simulink model "SolarTrackerVariantSubsystems"  (R2020a)
settings: Solver=FixedStepAuto  StartTime=0.0  StopTime=inf  RelTol=1e-3
model workspace (MAT data in the model file):
  readTSTime = 1
undefined symbols (not defined in the file): Fi, Wi
libraries: sldrtlib x9, arduinowifilib x5, simulink x4, arduinolib x2
settings Model: SILPILModeSetting=veronly  ExtModeTrigDuration=2  Creator=deepakbhatia  LastModifiedBy=cstapels
settings OptimizationCC: EnhancedBackFolding=on  PassReuseOutputArgsAs=Individual arguments  ZeroExternalMemoryAtStartup=off  ZeroInternalMemoryAtStartup=off  MaxStackSize=64  OptimizeBlockOrder=speed  DifferentSizesBufferReuse=on  OptimizationCustomize=off  EfficientTunableParamExpr=on
settings DebuggingCC: ParameterTunabilityLossMsg=error
settings HardwareCC: ProdBitPerPointer=32  ProdBitPerSizeT=32  ProdBitPerPtrDiffT=32  ProdLargestAtomicInteger=Long  ProdLargestAtomicFloat=Double  ProdWordSize=32  ProdHWDeviceType=ARM Compatible->ARM Cortex
settings SFSimCC: MATLABDynamicMemAlloc=off
settings RTWCC: SystemTargetFile=ert.tlc  HardwareBoard=Arduino MKR1000  TLCOptions=-aInlineSetEventsForThisBaseRateFcn=TLC_FALSE -aSuppressMultiTaskScheduler=TLC_FALSE -aRateBasedStepFcn=1  TemplateMakefile=ert_default_tmf  Toolchain=Arduino ARM  BuildConfiguration=Faster Runs
settings CodeAppCC: ForceParamTrailComments=on  IgnoreCustomStorageClasses=off  OperatorAnnotations=on  SimulinkDataObjDesc=on  SFDataObjDesc=on  InsertBlockDesc=on
settings ERTTargetCC: SupportContinuousTime=on  SupportVariableSizeSignals=on  ExtModeStaticAllocSize=8192

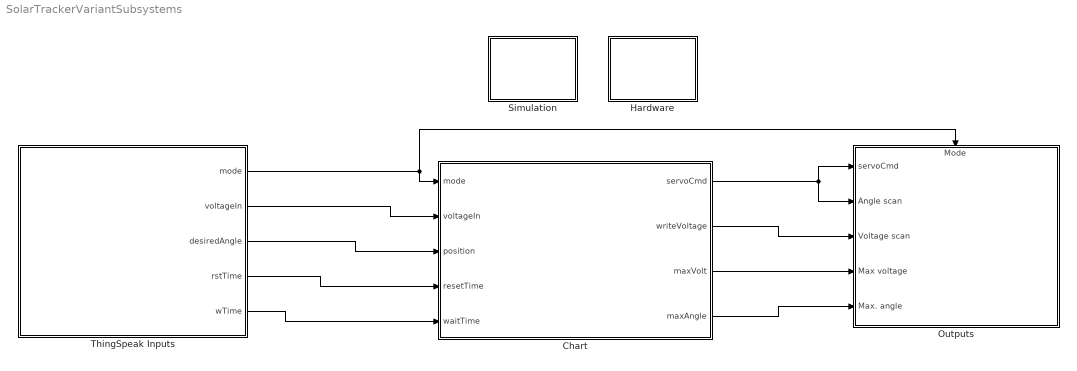
== system SolarTrackerVariantSubsystems ==
  Chart : Stateflow chart  TreatAsAtomicUnit=on
      settings: PortSchema="{\"entries\":[{\"content\":{\"sides\":[{\"content\":{\"connectorIds\":[\"In5\",\"In1\",\"In2\",\"In3\",\"In4\"]},\"type\":\"ConnectorPlacement.EquallySpacedRectSide\",\"uuid\":\"7460febf-f6e8-4dab-9ef6-8acf957c7b17\"},{\"content\":{\"connectorIds\":[\"Out1\",\"Out2\",\"Out3\",\"Out4\"],\"side\":\"RIGHT\"},\"type\":\"ConnectorPlacement.EquallySpacedRectSide\",\"uuid\":\"34f4fde0-3abd-4f83-b5ac-d115b7860e10\"},{\"content\":{\"connectorIds\":[],\"side\":\"TOP\"},\"type\":\"ConnectorPlacement.EquallySpacedRectSide\",\"uuid\":\"03c52414-b361-422d-a974-9760757eaedc\"}]},\"type\":\"ConnectorPlacement.EquallySpacedConnector\",\"uuid\":\"cf5b2fd0-3883-4494-a5b1-8c312db57bd7\"}],\"packageUris\":[\"http://schema.mathworks.com/mf0/Connector/19700101\"],\"version\":\"1.0\"}"
  Hardware : Subsystem
      settings: OpenFcn=|
      | simulationMode = 0
      | model = bdroot;
      | rtwbuild(model)
  Outputs : Subsystem  Variant=on
      settings: PortSchema="{\"entries\":[{\"content\":{\"sides\":[{\"content\":{\"connectorIds\":[\"In1\",\"In2\",\"In3\",\"In4\",\"In5\"]},\"type\":\"ConnectorPlacement.EquallySpacedRectSide\",\"uuid\":\"3daa0852-d339-48d5-aa09-9a267aadeaaa\"},{\"content\":{\"connectorIds\":[],\"side\":\"RIGHT\"},\"type\":\"ConnectorPlacement.EquallySpacedRectSide\",\"uuid\":\"98b05520-bee3-494f-8c4e-0b1eb9c00b10\"},{\"content\":{\"connectorIds\":[\"In6\"],\"side\":\"TOP\"},\"type\":\"ConnectorPlacement.EquallySpacedRectSide\",\"uuid\":\"246e7149-3295-4237-886d-aac11bde170e\"}]},\"type\":\"ConnectorPlacement.EquallySpacedConnector\",\"uuid\":\"0b2c3d1c-3ae1-45ce-8e4d-12c825df3e24\"}],\"packageUris\":[\"http://schema.mathworks.com/mf0/Connector/19700101\"],\"version\":\"1.0\"}"
  Simulation : Subsystem
      settings: OpenFcn=|
      | simulationMode = 1;
      | model=bdroot;
      | set_param(model,'SimulationCommand','start');
  ThingSpeak Inputs : Subsystem  Variant=on
  wires:
  ThingSpeak Inputs/2(voltageIn) -> Chart/1(voltageIn)
  ThingSpeak Inputs/4(rstTime) -> Chart/3(resetTime)
  ThingSpeak Inputs/5(wTime) -> Chart/4(waitTime)
  Chart/4(maxAngle) -> Outputs/5(Max. angle)
  ThingSpeak Inputs/1(mode) -> Chart/5(mode), Outputs/6(Mode)
  Chart/2(writeVoltage) -> Outputs/3(Voltage scan)
  Chart/1(servoCmd) -> Outputs/1(servoCmd), Outputs/2(Angle scan)
  Chart/3(maxVolt) -> Outputs/4(Max voltage)
  ThingSpeak Inputs/3(desiredAngle) -> Chart/2(position)

== system SolarTrackerVariantSubsystems/Hardware ==

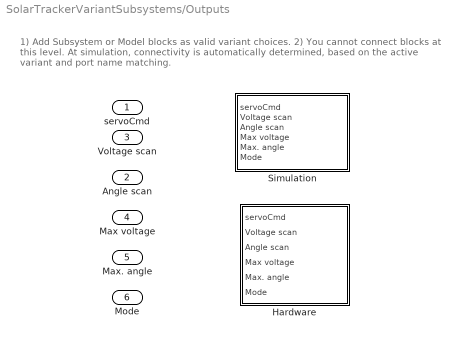
== system SolarTrackerVariantSubsystems/Outputs ==
  note: 1) Add Subsystem or Model blocks as valid variant choices.
      | 2) You cannot connect blocks at this level. At simulation, connectivity is automatically
      | determined, based on the active variant and port name matching.
  servoCmd : Inport
  Angle scan : Inport  Port=2
  Voltage scan : Inport  Port=3
  Max voltage : Inport  Port=4
  Max. angle : Inport  Port=5
  Mode : Inport  Port=6
  Hardware : Subsystem  VariantControl=simulationMode == 0
  Simulation : Subsystem  VariantControl=simulationMode == 1

== system SolarTrackerVariantSubsystems/Simulation ==

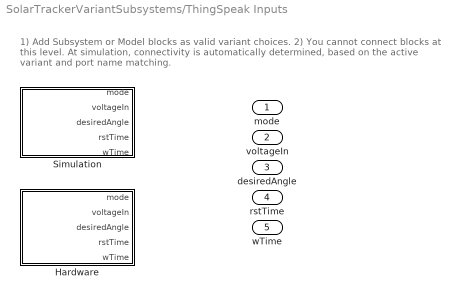
== system SolarTrackerVariantSubsystems/ThingSpeak Inputs ==
  note: 1) Add Subsystem or Model blocks as valid variant choices.
      | 2) You cannot connect blocks at this level. At simulation, connectivity is automatically
      | determined, based on the active variant and port name matching.
  Hardware : Subsystem  VariantControl=simulationMode == 0
  Simulation : Subsystem  VariantControl=simulationMode == 1
  mode : Outport
  voltageIn : Outport  Port=2
  desiredAngle : Outport  Port=3
  rstTime : Outport  Port=4
  wTime : Outport  Port=5

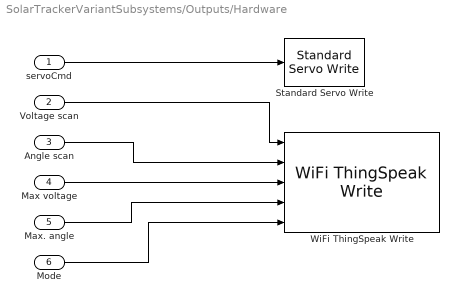
== system SolarTrackerVariantSubsystems/Outputs/Hardware ==
  servoCmd : Inport
  Voltage scan : Inport  Port=2
  Angle scan : Inport  Port=3
  Max voltage : Inport  Port=4
  Max. angle : Inport  Port=5
  Mode : Inport  Port=6
  Standard Servo Write : arduinolib/Standard Servo Write  pinNumber=9  ServoIndex=0  blockPlatform=ARDUINO
  WiFi ThingSpeak Write : arduinowifilib/WiFi ThingSpeak Write  ChannelID_=1049171  WriteAPIKey_=MXTVN2YNFBXXKHG7  NumberOfFields=5  UpdateInterval_=3  PrintDiagnosticMessages_=off  LocationEnabled=off  LocationSource=Block dialog  blockPlatform=arduino  Interfacetype_=Wi-Fi  UpdateURL=0  StatusMessage=0  StatusEnabled=on  StatusSource=<empty>
      settings: SourceProductBaseCode=ARDUINO
  wires:
  Voltage scan/1 -> WiFi ThingSpeak Write/1
  servoCmd/1 -> Standard Servo Write/1
  Max. angle/1 -> WiFi ThingSpeak Write/4
  Angle scan/1 -> WiFi ThingSpeak Write/2
  Mode/1 -> WiFi ThingSpeak Write/5
  Max voltage/1 -> WiFi ThingSpeak Write/3

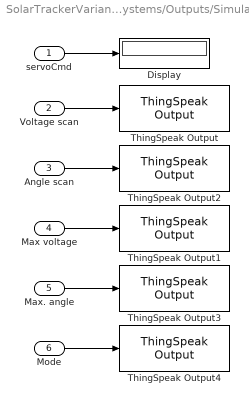
== system SolarTrackerVariantSubsystems/Outputs/Simulation ==
  servoCmd : Inport
  Voltage scan : Inport  Port=2
  Angle scan : Inport  Port=3
  Max voltage : Inport  Port=4
  Max. angle : Inport  Port=5
  Mode : Inport  Port=6
  Display : Display
  ThingSpeak Output : sldrtlib/Internet of Things/ThingSpeak Output  DrvAddress=1049171  DrvOptions=[1 10 77 88 84 86 78 50 89 78 70 66 88 88 75 72 71 55 97 112 105 46 116 104 105 110 103 115 112 101 97 107 46 99 111 109 0 0 0 0 0 0 0 0 0 0 0 0 0 0 0 0 0 0 0 0 0 0 0 0 0 0 0 0 0 0 0 0 0 0 0 0 0 0 0 0 0 0 0 0 0 0 0 0 0 0 0 0 0 0 0 0 0 0 0 0 0 0 0 0 0 0 0 0 0 0 0 0 0 0 0 0 0 0 0 0 0 0 0 0 0 0 0 0 0 0 0 0 0 0 0 0 0 0 0 0 0 0 0 0 0 0 0 0 0 0 0 0 0 0 0 0 0 0 0 0 0 0 0 0 0 0 0 0 0 0 0 0 0 0 0 0 0 0 0 0 0 0 0 0 0 0 0 0 0 0 0 0 0 0 0 0 0 0 0 0 0 0 0 0 0 0 0 0 0 0 0 0 0 0 0 0 0 0 0 0 0 0 0 0 0 0 0 0 0 0 0 0 0 0 0 0 0 0 0 0 0 0 0 0 0 0 0 0 0 0 0 0 0 0 0 0 0 0 0 0]  SampleTime=1  MaxMissedTicks=10  ShowMissedTicks=off  YieldWhenWaiting=off  ChannelFields=1  OptParam=0  InitialValue=[]  FinalValue=[]
      settings: SourceProductBaseCode=WT
  ThingSpeak Output1 : sldrtlib/Internet of Things/ThingSpeak Output  DrvAddress=1049171  DrvOptions=[1 10 77 88 84 86 78 50 89 78 70 66 88 88 75 72 71 55 97 112 105 46 116 104 105 110 103 115 112 101 97 107 46 99 111 109 0 0 0 0 0 0 0 0 0 0 0 0 0 0 0 0 0 0 0 0 0 0 0 0 0 0 0 0 0 0 0 0 0 0 0 0 0 0 0 0 0 0 0 0 0 0 0 0 0 0 0 0 0 0 0 0 0 0 0 0 0 0 0 0 0 0 0 0 0 0 0 0 0 0 0 0 0 0 0 0 0 0 0 0 0 0 0 0 0 0 0 0 0 0 0 0 0 0 0 0 0 0 0 0 0 0 0 0 0 0 0 0 0 0 0 0 0 0 0 0 0 0 0 0 0 0 0 0 0 0 0 0 0 0 0 0 0 0 0 0 0 0 0 0 0 0 0 0 0 0 0 0 0 0 0 0 0 0 0 0 0 0 0 0 0 0 0 0 0 0 0 0 0 0 0 0 0 0 0 0 0 0 0 0 0 0 0 0 0 0 0 0 0 0 0 0 0 0 0 0 0 0 0 0 0 0 0 0 0 0 0 0 0 0 0 0 0 0 0 0]  SampleTime=1  MaxMissedTicks=10  ShowMissedTicks=off  YieldWhenWaiting=off  ChannelFields=3  OptParam=0  InitialValue=[]  FinalValue=[]
      settings: SourceProductBaseCode=WT
  ThingSpeak Output2 : sldrtlib/Internet of Things/ThingSpeak Output  DrvAddress=1049171  DrvOptions=[1 10 77 88 84 86 78 50 89 78 70 66 88 88 75 72 71 55 97 112 105 46 116 104 105 110 103 115 112 101 97 107 46 99 111 109 0 0 0 0 0 0 0 0 0 0 0 0 0 0 0 0 0 0 0 0 0 0 0 0 0 0 0 0 0 0 0 0 0 0 0 0 0 0 0 0 0 0 0 0 0 0 0 0 0 0 0 0 0 0 0 0 0 0 0 0 0 0 0 0 0 0 0 0 0 0 0 0 0 0 0 0 0 0 0 0 0 0 0 0 0 0 0 0 0 0 0 0 0 0 0 0 0 0 0 0 0 0 0 0 0 0 0 0 0 0 0 0 0 0 0 0 0 0 0 0 0 0 0 0 0 0 0 0 0 0 0 0 0 0 0 0 0 0 0 0 0 0 0 0 0 0 0 0 0 0 0 0 0 0 0 0 0 0 0 0 0 0 0 0 0 0 0 0 0 0 0 0 0 0 0 0 0 0 0 0 0 0 0 0 0 0 0 0 0 0 0 0 0 0 0 0 0 0 0 0 0 0 0 0 0 0 0 0 0 0 0 0 0 0 0 0 0 0 0 0]  SampleTime=1  MaxMissedTicks=10  ShowMissedTicks=off  YieldWhenWaiting=off  ChannelFields=2  OptParam=0  InitialValue=[]  FinalValue=[]
      settings: SourceProductBaseCode=WT
  ThingSpeak Output3 : sldrtlib/Internet of Things/ThingSpeak Output  DrvAddress=1049171  DrvOptions=[1 10 77 88 84 86 78 50 89 78 70 66 88 88 75 72 71 55 97 112 105 46 116 104 105 110 103 115 112 101 97 107 46 99 111 109 0 0 0 0 0 0 0 0 0 0 0 0 0 0 0 0 0 0 0 0 0 0 0 0 0 0 0 0 0 0 0 0 0 0 0 0 0 0 0 0 0 0 0 0 0 0 0 0 0 0 0 0 0 0 0 0 0 0 0 0 0 0 0 0 0 0 0 0 0 0 0 0 0 0 0 0 0 0 0 0 0 0 0 0 0 0 0 0 0 0 0 0 0 0 0 0 0 0 0 0 0 0 0 0 0 0 0 0 0 0 0 0 0 0 0 0 0 0 0 0 0 0 0 0 0 0 0 0 0 0 0 0 0 0 0 0 0 0 0 0 0 0 0 0 0 0 0 0 0 0 0 0 0 0 0 0 0 0 0 0 0 0 0 0 0 0 0 0 0 0 0 0 0 0 0 0 0 0 0 0 0 0 0 0 0 0 0 0 0 0 0 0 0 0 0 0 0 0 0 0 0 0 0 0 0 0 0 0 0 0 0 0 0 0 0 0 0 0 0 0]  SampleTime=1  MaxMissedTicks=10  ShowMissedTicks=off  YieldWhenWaiting=off  ChannelFields=4  OptParam=0  InitialValue=[]  FinalValue=[]
      settings: SourceProductBaseCode=WT
  ThingSpeak Output4 : sldrtlib/Internet of Things/ThingSpeak Output  DrvAddress=1049171  DrvOptions=[1 10 77 88 84 86 78 50 89 78 70 66 88 88 75 72 71 55 97 112 105 46 116 104 105 110 103 115 112 101 97 107 46 99 111 109 0 0 0 0 0 0 0 0 0 0 0 0 0 0 0 0 0 0 0 0 0 0 0 0 0 0 0 0 0 0 0 0 0 0 0 0 0 0 0 0 0 0 0 0 0 0 0 0 0 0 0 0 0 0 0 0 0 0 0 0 0 0 0 0 0 0 0 0 0 0 0 0 0 0 0 0 0 0 0 0 0 0 0 0 0 0 0 0 0 0 0 0 0 0 0 0 0 0 0 0 0 0 0 0 0 0 0 0 0 0 0 0 0 0 0 0 0 0 0 0 0 0 0 0 0 0 0 0 0 0 0 0 0 0 0 0 0 0 0 0 0 0 0 0 0 0 0 0 0 0 0 0 0 0 0 0 0 0 0 0 0 0 0 0 0 0 0 0 0 0 0 0 0 0 0 0 0 0 0 0 0 0 0 0 0 0 0 0 0 0 0 0 0 0 0 0 0 0 0 0 0 0 0 0 0 0 0 0 0 0 0 0 0 0 0 0 0 0 0 0]  SampleTime=1  MaxMissedTicks=10  ShowMissedTicks=off  YieldWhenWaiting=off  ChannelFields=5  OptParam=0  InitialValue=[]  FinalValue=[]
      settings: SourceProductBaseCode=WT
  wires:
  Mode/1 -> ThingSpeak Output4/1
  Voltage scan/1 -> ThingSpeak Output/1
  Max voltage/1 -> ThingSpeak Output1/1
  Max. angle/1 -> ThingSpeak Output3/1
  Angle scan/1 -> ThingSpeak Output2/1
  servoCmd/1 -> Display/1

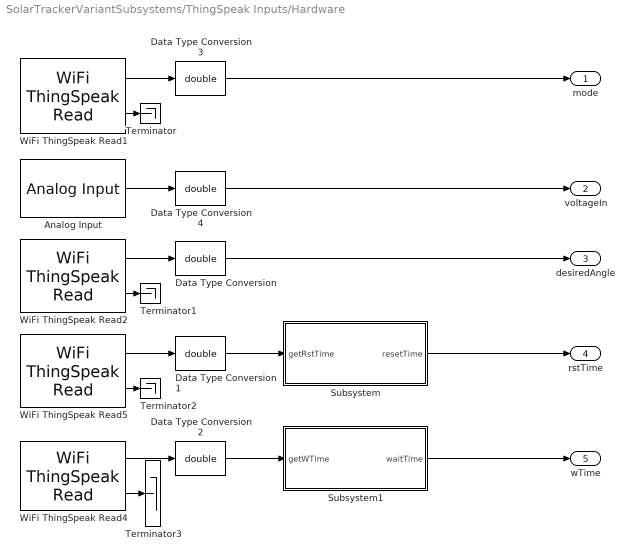
== system SolarTrackerVariantSubsystems/ThingSpeak Inputs/Hardware ==
  Analog Input : arduinolib/Analog Input  pinNumber=1  ReadResultsOnly=off  ConversionTriggerSource=Software  ExternalTriggerType=uint32( 0 )  OutputDataType=uint16  EnableConversionCompleteNotify=off  EnableOuputStatus=off  SampleTime=-1  blockPlatform=arduino
      settings: AttributesFormatString=Input Voltage
  Data Type Conversion{,1..4} (5 alike) : DataTypeConversion  OutDataTypeStr=double
  Subsystem : Subsystem
  Subsystem1 : Subsystem
  Terminator{,1..3} (4 alike) : Terminator
  WiFi ThingSpeak Read1 : arduinowifilib/WiFi ThingSpeak Read  ChannelID_=1005403  ChannelAccess_=Private  ReadAPIKey_=RTAKGVYMGG3OII72  FieldNumber_=1  PrintDiagnosticMessages_=off  blockPlatform=Arduino  Interfacetype_=Wi-Fi  SampleTime_=30
      settings: AttributesFormatString=Mode Select  SourceProductBaseCode=ARDUINO
  WiFi ThingSpeak Read2 : arduinowifilib/WiFi ThingSpeak Read  ChannelID_=1005403  ChannelAccess_=Private  ReadAPIKey_=RTAKGVYMGG3OII72  FieldNumber_=2  PrintDiagnosticMessages_=off  blockPlatform=Arduino  Interfacetype_=Wi-Fi  SampleTime_=30
      settings: AttributesFormatString=Desired Position  SourceProductBaseCode=ARDUINO
  WiFi ThingSpeak Read4 : arduinowifilib/WiFi ThingSpeak Read  ChannelID_=1005403  ChannelAccess_=Private  ReadAPIKey_=RTAKGVYMGG3OII72  FieldNumber_=4  PrintDiagnosticMessages_=off  blockPlatform=Arduino  Interfacetype_=Wi-Fi  SampleTime_=30
      settings: AttributesFormatString=Wait Time  SourceProductBaseCode=ARDUINO
  WiFi ThingSpeak Read5 : arduinowifilib/WiFi ThingSpeak Read  ChannelID_=1005403  ChannelAccess_=Private  ReadAPIKey_=RTAKGVYMGG3OII72  FieldNumber_=3  PrintDiagnosticMessages_=off  blockPlatform=Arduino  Interfacetype_=Wi-Fi  SampleTime_=30
      settings: AttributesFormatString=Reset Time  SourceProductBaseCode=ARDUINO
  mode : Outport
  voltageIn : Outport  Port=2
  desiredAngle : Outport  Port=3
  rstTime : Outport  Port=4
  wTime : Outport  Port=5
  wires:
  Data Type Conversion2/1 -> Subsystem1/1(getWTime)
  WiFi ThingSpeak Read1/2 -> Terminator/1
  WiFi ThingSpeak Read2/1 -> Data Type Conversion/1
  WiFi ThingSpeak Read1/1 -> Data Type Conversion3/1
  Data Type Conversion1/1 -> Subsystem/1(getRstTime)
  WiFi ThingSpeak Read2/2 -> Terminator1/1
  Data Type Conversion4/1 -> voltageIn/1
  WiFi ThingSpeak Read5/2 -> Terminator2/1
  WiFi ThingSpeak Read4/1 -> Data Type Conversion2/1
  WiFi ThingSpeak Read5/1 -> Data Type Conversion1/1
  WiFi ThingSpeak Read4/2 -> Terminator3/1
  Data Type Conversion/1 -> desiredAngle/1
  Analog Input/1 -> Data Type Conversion4/1
  Data Type Conversion3/1 -> mode/1
  Subsystem1/1(waitTime) -> wTime/1
  Subsystem/1(resetTime) -> rstTime/1

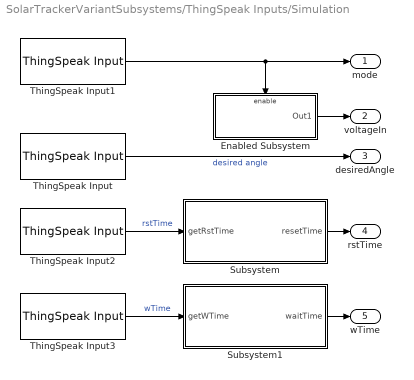
== system SolarTrackerVariantSubsystems/ThingSpeak Inputs/Simulation ==
  Enabled Subsystem : Subsystem  TreatAsAtomicUnit=on
  Subsystem : Subsystem
  Subsystem1 : Subsystem
  ThingSpeak Input : sldrtlib/Internet of Things/ThingSpeak Input  DrvAddress=1049139  DrvOptions=[0 1 84 52 67 75 85 73 73 71 66 66 69 84 80 70 66 68 97 112 105 46 116 104 105 110 103 115 112 101 97 107 46 99 111 109 0 0 0 0 0 0 0 0 0 0 0 0 0 0 0 0 0 0 0 0 0 0 0 0 0 0 0 0 0 0 0 0 0 0 0 0 0 0 0 0 0 0 0 0 0 0 0 0 0 0 0 0 0 0 0 0 0 0 0 0 0 0 0 0 0 0 0 0 0 0 0 0 0 0 0 0 0 0 0 0 0 0 0 0 0 0 0 0 0 0 0 0 0 0 0 0 0 0 0 0 0 0 0 0 0 0 0 0 0 0 0 0 0 0 0 0 0 0 0 0 0 0 0 0 0 0 0 0 0 0 0 0 0 0 0 0 0 0 0 0 0 0 0 0 0 0 0 0 0 0 0 0 0 0 0 0 0 0 0 0 0 0 0 0 0 0 0 0 0 0 0 0 0 0 0 0 0 0 0 0 0 0 0 0 0 0 0 0 0 0 0 0 0 0 0 0 0 0 0 0 0 0 0 0 0 0 0 0 0 0 0 0 0 0 0 0 0 0 0 0]  SampleTime=1  MaxMissedTicks=10  ShowMissedTicks=off  YieldWhenWaiting=off  ChannelFields=2  OptParam=0  DataTypeStr=double
      settings: AttributesFormatString=Desired Angle  SourceProductBaseCode=WT
  ThingSpeak Input1 : sldrtlib/Internet of Things/ThingSpeak Input  DrvAddress=1049139  DrvOptions=[0 1 84 52 67 75 85 73 73 71 66 66 69 84 80 70 66 68 97 112 105 46 116 104 105 110 103 115 112 101 97 107 46 99 111 109 0 0 0 0 0 0 0 0 0 0 0 0 0 0 0 0 0 0 0 0 0 0 0 0 0 0 0 0 0 0 0 0 0 0 0 0 0 0 0 0 0 0 0 0 0 0 0 0 0 0 0 0 0 0 0 0 0 0 0 0 0 0 0 0 0 0 0 0 0 0 0 0 0 0 0 0 0 0 0 0 0 0 0 0 0 0 0 0 0 0 0 0 0 0 0 0 0 0 0 0 0 0 0 0 0 0 0 0 0 0 0 0 0 0 0 0 0 0 0 0 0 0 0 0 0 0 0 0 0 0 0 0 0 0 0 0 0 0 0 0 0 0 0 0 0 0 0 0 0 0 0 0 0 0 0 0 0 0 0 0 0 0 0 0 0 0 0 0 0 0 0 0 0 0 0 0 0 0 0 0 0 0 0 0 0 0 0 0 0 0 0 0 0 0 0 0 0 0 0 0 0 0 0 0 0 0 0 0 0 0 0 0 0 0 0 0 0 0 0 0]  SampleTime=1  MaxMissedTicks=10  ShowMissedTicks=off  YieldWhenWaiting=off  ChannelFields=1  OptParam=0  DataTypeStr=double
      settings: AttributesFormatString=Mode Select  SourceProductBaseCode=WT
  ThingSpeak Input2 : sldrtlib/Internet of Things/ThingSpeak Input  DrvAddress=1049139  DrvOptions=[0 1 84 52 67 75 85 73 73 71 66 66 69 84 80 70 66 68 97 112 105 46 116 104 105 110 103 115 112 101 97 107 46 99 111 109 0 0 0 0 0 0 0 0 0 0 0 0 0 0 0 0 0 0 0 0 0 0 0 0 0 0 0 0 0 0 0 0 0 0 0 0 0 0 0 0 0 0 0 0 0 0 0 0 0 0 0 0 0 0 0 0 0 0 0 0 0 0 0 0 0 0 0 0 0 0 0 0 0 0 0 0 0 0 0 0 0 0 0 0 0 0 0 0 0 0 0 0 0 0 0 0 0 0 0 0 0 0 0 0 0 0 0 0 0 0 0 0 0 0 0 0 0 0 0 0 0 0 0 0 0 0 0 0 0 0 0 0 0 0 0 0 0 0 0 0 0 0 0 0 0 0 0 0 0 0 0 0 0 0 0 0 0 0 0 0 0 0 0 0 0 0 0 0 0 0 0 0 0 0 0 0 0 0 0 0 0 0 0 0 0 0 0 0 0 0 0 0 0 0 0 0 0 0 0 0 0 0 0 0 0 0 0 0 0 0 0 0 0 0 0 0 0 0 0 0]  SampleTime=1  MaxMissedTicks=10  ShowMissedTicks=off  YieldWhenWaiting=off  ChannelFields=3  OptParam=0  DataTypeStr=double
      settings: AttributesFormatString=Reset Time  SourceProductBaseCode=WT
  ThingSpeak Input3 : sldrtlib/Internet of Things/ThingSpeak Input  DrvAddress=1049139  DrvOptions=[0 1 84 52 67 75 85 73 73 71 66 66 69 84 80 70 66 68 97 112 105 46 116 104 105 110 103 115 112 101 97 107 46 99 111 109 0 0 0 0 0 0 0 0 0 0 0 0 0 0 0 0 0 0 0 0 0 0 0 0 0 0 0 0 0 0 0 0 0 0 0 0 0 0 0 0 0 0 0 0 0 0 0 0 0 0 0 0 0 0 0 0 0 0 0 0 0 0 0 0 0 0 0 0 0 0 0 0 0 0 0 0 0 0 0 0 0 0 0 0 0 0 0 0 0 0 0 0 0 0 0 0 0 0 0 0 0 0 0 0 0 0 0 0 0 0 0 0 0 0 0 0 0 0 0 0 0 0 0 0 0 0 0 0 0 0 0 0 0 0 0 0 0 0 0 0 0 0 0 0 0 0 0 0 0 0 0 0 0 0 0 0 0 0 0 0 0 0 0 0 0 0 0 0 0 0 0 0 0 0 0 0 0 0 0 0 0 0 0 0 0 0 0 0 0 0 0 0 0 0 0 0 0 0 0 0 0 0 0 0 0 0 0 0 0 0 0 0 0 0 0 0 0 0 0 0]  SampleTime=1  MaxMissedTicks=10  ShowMissedTicks=off  YieldWhenWaiting=off  ChannelFields=4  OptParam=0  DataTypeStr=double
      settings: AttributesFormatString=Wait Time  SourceProductBaseCode=WT
  mode : Outport
  voltageIn : Outport  Port=2
  desiredAngle : Outport  Port=3
  rstTime : Outport  Port=4
  wTime : Outport  Port=5
  wires:
  ThingSpeak Input1/1 -> mode/1, Enabled Subsystem/Enable
  ThingSpeak Input3/1 -> Subsystem1/1(getWTime)  "wTime"
  Subsystem1/1(waitTime) -> wTime/1
  Enabled Subsystem/1(Out1) -> voltageIn/1
  ThingSpeak Input2/1 -> Subsystem/1(getRstTime)  "rstTime"
  ThingSpeak Input/1 -> desiredAngle/1  "desired angle"
  Subsystem/1(resetTime) -> rstTime/1

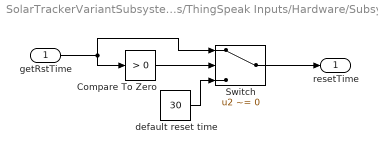
== system SolarTrackerVariantSubsystems/ThingSpeak Inputs/Hardware/Subsystem ==
  getRstTime : Inport  OutDataTypeStr=double
  Compare To Zero : simulink/Logic and Bit Operations/Compare To Zero  relop=>  OutDataTypeStr=boolean
  Switch : Switch  Criteria=u2 ~= 0
  default reset time : Constant  Value=30  SampleTime=-1
  resetTime : Outport  OutDataTypeStr=double
  wires:
  Compare To Zero/1 -> Switch/2
  default reset time/1 -> Switch/3
  getRstTime/1 -> Switch/1, Compare To Zero/1
  Switch/1 -> resetTime/1

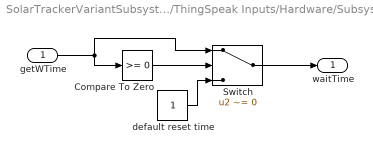
== system SolarTrackerVariantSubsystems/ThingSpeak Inputs/Hardware/Subsystem1 ==
  getWTime : Inport  OutDataTypeStr=double
  Compare To Zero : simulink/Logic and Bit Operations/Compare To Zero  relop=>=  OutDataTypeStr=boolean
  Switch : Switch  Criteria=u2 ~= 0  OutDataTypeStr=double
  default reset time : Constant  SampleTime=-1
  waitTime : Outport  OutDataTypeStr=double
  wires:
  Compare To Zero/1 -> Switch/2
  default reset time/1 -> Switch/3
  getWTime/1 -> Switch/1, Compare To Zero/1
  Switch/1 -> waitTime/1

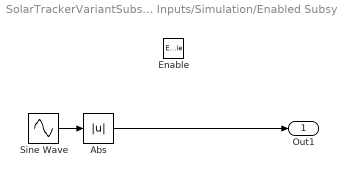
== system SolarTrackerVariantSubsystems/ThingSpeak Inputs/Simulation/Enabled Subsystem ==
  Enable : EnablePort  StatesWhenEnabling=reset
  Abs : Abs
  Sine Wave : Sin  Amplitude=3.4  Frequency=0.01  SampleTime=1
  Out1 : Outport
  wires:
  Abs/1 -> Out1/1
  Sine Wave/1 -> Abs/1

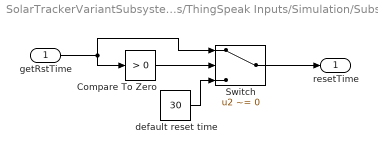
== system SolarTrackerVariantSubsystems/ThingSpeak Inputs/Simulation/Subsystem ==
  getRstTime : Inport  OutDataTypeStr=double
  Compare To Zero : simulink/Logic and Bit Operations/Compare To Zero  relop=>  OutDataTypeStr=boolean
  Switch : Switch  Criteria=u2 ~= 0
  default reset time : Constant  Value=30  SampleTime=1
  resetTime : Outport  OutDataTypeStr=double
  wires:
  Compare To Zero/1 -> Switch/2
  default reset time/1 -> Switch/3
  getRstTime/1 -> Switch/1, Compare To Zero/1
  Switch/1 -> resetTime/1

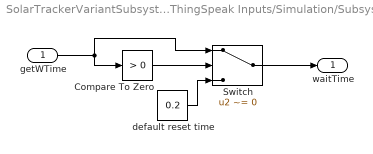
== system SolarTrackerVariantSubsystems/ThingSpeak Inputs/Simulation/Subsystem1 ==
  getWTime : Inport  OutDataTypeStr=double
  Compare To Zero : simulink/Logic and Bit Operations/Compare To Zero  relop=>  OutDataTypeStr=boolean
  Switch : Switch  Criteria=u2 ~= 0  OutDataTypeStr=Inherit: Inherit via back propagation
  default reset time : Constant  Value=0.2  SampleTime=1
  waitTime : Outport  OutDataTypeStr=double
  wires:
  Compare To Zero/1 -> Switch/2
  default reset time/1 -> Switch/3
  getWTime/1 -> Switch/1, Compare To Zero/1
  Switch/1 -> waitTime/1

== stateflow chart SolarTrackerVariantSubsystems/Chart ==
  settings: updateMethod=DISCRETE  sampleTime=0.1
  state GoToPosition
    servoCmd = position;
    writeVoltage=voltageIn;
  state ScanAndGoToMaxVoltage
    state ResetPosition
      servoCmd = 0;
      voltage = zeros(1,181);
    state ScanVoltages
      servoCmd = angleRange(i);
      voltage(i) = voltageIn;
      writeVoltage = voltage(i);
    state Increment
      entry: i = i + 5;
    state GoToMaxVoltage
      [maxVolt,maxVoltAngle] = max(voltage);
      servoCmd = angleRange(maxVoltAngle);
      maxAngle = servoCmd;
      writeVoltage=voltageIn;
    (default) -> ResetPosition : {angleRange = 0 :180;}
    GoToMaxVoltage -> ResetPosition : after(resetTime,sec)
    ResetPosition -> ScanVoltages : {i = 1;}
    ScanVoltages -> Increment [order 1] : [i < 181]
    Increment -> ScanVoltages : after(waitTime,msec)
    ScanVoltages -> GoToMaxVoltage [order 2] : [i==181]
  (default) -> GoToPosition
  GoToPosition -> ScanAndGoToMaxVoltage : [mode==1]
  ScanAndGoToMaxVoltage -> GoToPosition : [mode==0]
  data: voltageIn input; position input; servoCmd output; writeVoltage output; maxVolt output; maxAngle output; voltage local; i local; maxVoltAngle local; resetTime input; waitTime input; mode input; angleRange local
